simulink model "SimulateBatteryModel"  (R2018a)
settings: Solver=FixedStepAuto  StartTime=0.0  StopTime=50000  FixedStep=0.015  RelTol=1e-3  EnableMultiTasking=on
values from neighbouring files (symbols this model uses):
  charge_current = -20    [BatteryTest.m]
  charge_switch = 0    [BatteryTest.m]
  discharge_current = 20    [BatteryTest.m]
undefined symbols (not defined in the file or in its folder): Ion, Li
libraries: simulink x4, Lib_PB_Battery_TMATS x1
settings Model: Creator=ewong  LastModifiedBy=mebell
settings OptimizationCC: LifeSpan=inf
settings DebuggingCC: SFUnexpectedBacktrackingDiag=warning  SFNoUnconditionalDefaultTransitionDiag=warning  SFExecutionAtInitializationDiag=none
settings CodeAppCC: StateflowObjectComments=on
settings GRTTargetCC: TargetLangStandard=C89/C90 (ANSI)  GeneratePreprocessorConditionals=Disable all
settings ConfigComp: CovMetricSettings=dw  CovHtmlReporting=on  CovSaveCumulativeToWorkspaceVar=on  CovSaveSingleToWorkspaceVar=on  CovExternalEMLEnable=off

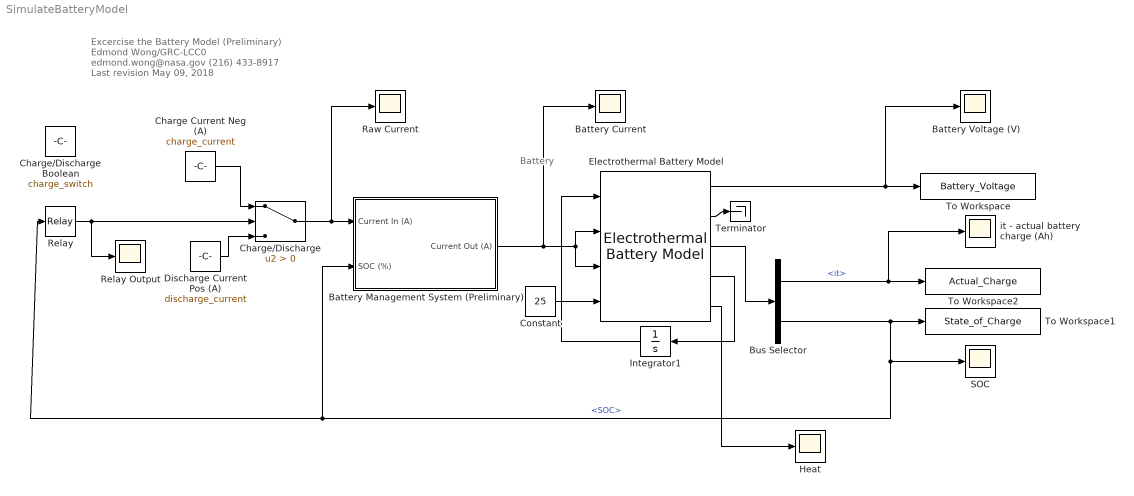
== system SimulateBatteryModel ==
  note: Excercise the Battery Model (Preliminary)
      | Edmond Wong/GRC-LCC0
      | edmond.wong@nasa.gov
      | (216) 433-8917
      |
      | Last revision May 09, 2018
  note: Battery
  Battery Current : Scope
  Battery Management System (Preliminary) : Subsystem
  Battery Voltage (V) : Scope
  Bus Selector : BusSelector  OutputSignals=it,SOC
  Charge Current Neg (A) : Constant  Value=charge_current
  Charge/Discharge : Switch  Criteria=u2 > Threshold
  Charge/Discharge Boolean : Constant  Value=charge_switch  OutDataTypeStr=boolean
  Constant : Constant  Value=25
  Discharge Current Pos (A) : Constant  Value=discharge_current
  "Electrothermal Battery Model " : Lib_PB_Battery_TMATS/Electrothermal Battery Model   E0_M=3.3  Q_M=Q  R_M=R  K_M=K  B_M=B  SOC_Init_M=100.0  A_M=A  battery_type_M=Li-Ion  TempIn=Celsius
  Heat : Scope
  Integrator1 : Integrator
  Raw Current : Scope
  Relay : Relay  OnSwitchValue=99  OffSwitchValue=3  OnOutputValue=0  OffOutputValue=5
  Relay Output : Scope
  SOC : Scope
  Terminator : Terminator
  To Workspace : ToWorkspace  VariableName=Battery_Voltage  SampleTime=-1
  To Workspace1 : ToWorkspace  VariableName=State_of_Charge  SampleTime=-1
  To Workspace2 : ToWorkspace  VariableName=Actual_Charge  SampleTime=-1
  it - actual battery charge (Ah) : Scope
  wires:
  Discharge Current Pos (A)/1 -> Charge/Discharge/3
  Charge Current Neg (A)/1 -> Charge/Discharge/1
  Relay/1 -> Relay Output/1, Charge/Discharge/2
  Bus Selector/2 -> Battery Management System (Preliminary)/2(SOC (%)), Relay/1, SOC/1, To Workspace1/1  "<SOC>"
  "Electrothermal Battery Model "/1 -> Battery Voltage (V)/1, To Workspace/1
  Integrator1/1 -> "Electrothermal Battery Model "/1
  Charge/Discharge/1 -> Raw Current/1, Battery Management System (Preliminary)/1(Current In (A))
  Battery Management System (Preliminary)/1(Current Out (A)) -> "Electrothermal Battery Model "/2, "Electrothermal Battery Model "/3, Battery Current/1
  Bus Selector/1 -> it - actual battery charge (Ah)/1, To Workspace2/1  "<it>"
  "Electrothermal Battery Model "/3 -> Bus Selector/1
  "Electrothermal Battery Model "/4 -> Integrator1/1
  "Electrothermal Battery Model "/2 -> Terminator/1
  "Electrothermal Battery Model "/5 -> Heat/1
  Constant/1 -> "Electrothermal Battery Model "/4

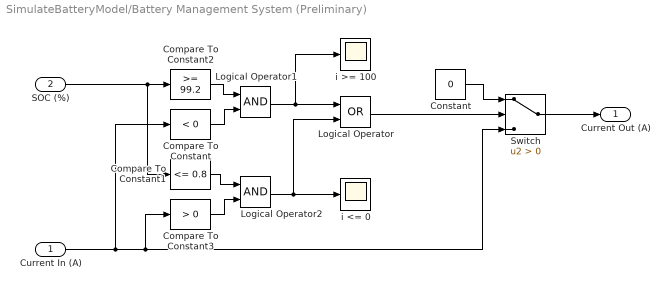
== system SimulateBatteryModel/Battery Management System (Preliminary) ==
  Current In (A) : Inport
  SOC (%) : Inport  Port=2
  Compare To Constant : simulink/Logic and Bit Operations/Compare To Constant  relop=<  const=0  OutDataTypeStr=boolean
  Compare To Constant1 : simulink/Logic and Bit Operations/Compare To Constant  relop=<=  const=0.8  OutDataTypeStr=boolean
  Compare To Constant2 : simulink/Logic and Bit Operations/Compare To Constant  relop=>=  const=99.2  OutDataTypeStr=boolean
  Compare To Constant3 : simulink/Logic and Bit Operations/Compare To Constant  relop=>  const=0  OutDataTypeStr=boolean
  Constant : Constant  Value=0
  Logical Operator : Logic  Operator=OR  AllPortsSameDT=off  OutDataTypeStr=boolean
  Logical Operator1 : Logic  AllPortsSameDT=off  OutDataTypeStr=boolean
  Logical Operator2 : Logic  AllPortsSameDT=off  OutDataTypeStr=boolean
  Switch : Switch  Criteria=u2 > Threshold
  i <= 0 : Scope
  i >= 100 : Scope
  Current Out (A) : Outport
  wires:
  Constant/1 -> Switch/1
  Logical Operator/1 -> Switch/2
  Current In (A)/1 -> Compare To Constant/1, Compare To Constant3/1, Switch/3
  SOC (%)/1 -> Compare To Constant1/1, Compare To Constant2/1
  Compare To Constant2/1 -> Logical Operator1/1
  Compare To Constant/1 -> Logical Operator1/2
  Compare To Constant1/1 -> Logical Operator2/1
  Compare To Constant3/1 -> Logical Operator2/2
  Logical Operator1/1 -> i >= 100/1, Logical Operator/1
  Logical Operator2/1 -> i <= 0/1, Logical Operator/2
  Switch/1 -> Current Out (A)/1
